simulink model "PID_Gravity"  (R2024a)
settings: Solver=FixedStepAuto  StartTime=0.0  StopTime=10.0  FixedStep=1e-5  RelTol=1e-3
settings Model: Creator=erhan  LastModifiedBy=erhan

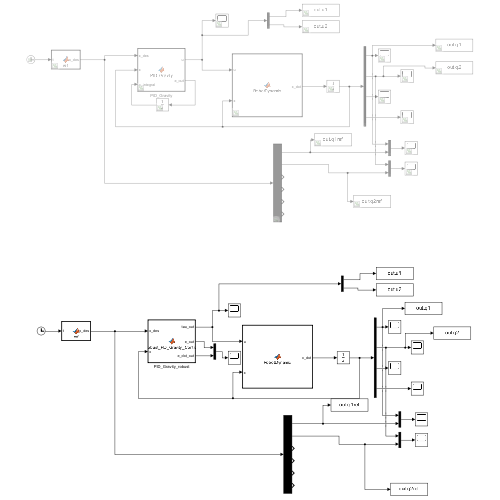
[thumbnail: Simulink's stored preview of the top-level diagram]
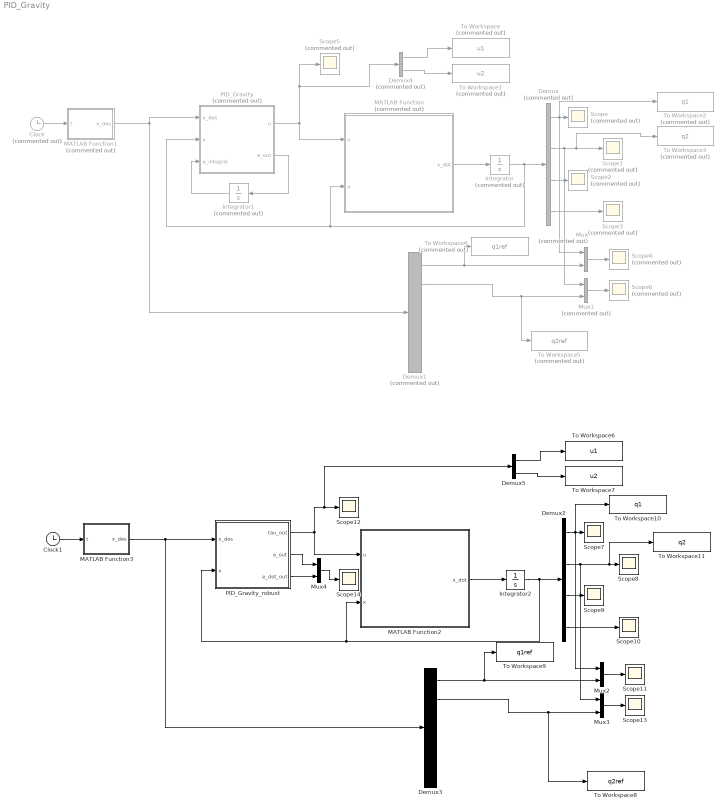
== system PID_Gravity ==
  Clock : Clock  Commented=on
  Clock1 : Clock
  Demux : Demux  Commented=on
  Demux1 : Demux  Commented=on  Outputs=6
  Demux2 : Demux
  Demux3 : Demux  Outputs=6
  Demux4 : Demux  Commented=on  Outputs=2
  Demux5 : Demux  Outputs=2
  Integrator : Integrator  Commented=on  InitialCondition=[0;0;0;0]
  Integrator1 : Integrator  Commented=on  InitialCondition=[0;0]
  Integrator2 : Integrator  InitialCondition=[0;0;0;0]
  MATLAB Function : MATLAB Function  Commented=on  TreatAsAtomicUnit=on
  MATLAB Function1 : MATLAB Function  Commented=on  TreatAsAtomicUnit=on
  MATLAB Function2 : MATLAB Function  TreatAsAtomicUnit=on
  MATLAB Function3 : MATLAB Function  TreatAsAtomicUnit=on
  Mux : Mux  Commented=on  Inputs=2
  Mux1 : Mux  Commented=on  Inputs=2
  Mux2 : Mux  Inputs=2
  Mux3 : Mux  Inputs=2
  Mux4 : Mux  Inputs=2
  PID_Gravity : MATLAB Function  Commented=on  TreatAsAtomicUnit=on
  PID_Gravity_robust : MATLAB Function  TreatAsAtomicUnit=on
  Scope{,1..6} (7 alike) : Scope  Commented=on
  Scope{7..14} (8 alike) : Scope
  To Workspace : ToWorkspace  Commented=on  VariableName=u1  SaveFormat=Timeseries  SampleTime=-1
  To Workspace1 : ToWorkspace  Commented=on  VariableName=u2  SaveFormat=Timeseries  SampleTime=-1
  To Workspace10 : ToWorkspace  VariableName=q1  SaveFormat=Timeseries  SampleTime=-1
  To Workspace11 : ToWorkspace  VariableName=q2  SaveFormat=Timeseries  SampleTime=-1
  To Workspace2 : ToWorkspace  Commented=on  VariableName=q1  SaveFormat=Timeseries  SampleTime=-1
  To Workspace3 : ToWorkspace  Commented=on  VariableName=q2  SaveFormat=Timeseries  SampleTime=-1
  To Workspace4 : ToWorkspace  Commented=on  VariableName=q1ref  SaveFormat=Timeseries  SampleTime=-1
  To Workspace5 : ToWorkspace  Commented=on  VariableName=q2ref  SaveFormat=Timeseries  SampleTime=-1
  To Workspace6 : ToWorkspace  VariableName=u1  SaveFormat=Timeseries  SampleTime=-1
  To Workspace7 : ToWorkspace  VariableName=u2  SaveFormat=Timeseries  SampleTime=-1
  To Workspace8 : ToWorkspace  VariableName=q2ref  SaveFormat=Timeseries  SampleTime=-1
  To Workspace9 : ToWorkspace  VariableName=q1ref  SaveFormat=Timeseries  SampleTime=-1
  wires:
  MATLAB Function/1(x_dot) -> Integrator/1
  Integrator/1 -> Demux/1, PID_Gravity/2(x), MATLAB Function/2(x)
  Demux/1 -> To Workspace2/1, Mux/1, Scope/1
  Demux/2 -> To Workspace3/1, Scope1/1, Mux1/1
  Demux/3 -> Scope2/1
  Demux/4 -> Scope3/1
  PID_Gravity/1(u) -> MATLAB Function/1(u), Demux4/1, Scope5/1
  MATLAB Function1/1(x_des) -> Demux1/1, PID_Gravity/1(x_des)
  Clock/1 -> MATLAB Function1/1(t)
  Mux/1 -> Scope4/1
  Demux1/1 -> To Workspace4/1, Mux/2
  Demux1/2 -> To Workspace5/1, Mux1/2
  Mux1/1 -> Scope6/1
  PID_Gravity/2(e_out) -> Integrator1/1
  Integrator1/1 -> PID_Gravity/3(e_integral)
  Mux3/1 -> Scope13/1
  Demux3/1 -> To Workspace9/1, Mux2/2
  Mux2/1 -> Scope11/1
  Clock1/1 -> MATLAB Function3/1(t)
  MATLAB Function3/1(x_des) -> PID_Gravity_robust/1(x_des), Demux3/1
  PID_Gravity_robust/1(tau_out) -> MATLAB Function2/1(u), Demux5/1, Scope12/1
  Demux2/4 -> Scope10/1
  Demux2/3 -> Scope9/1
  Demux2/2 -> Mux3/1, To Workspace11/1, Scope8/1
  Demux2/1 -> To Workspace10/1, Scope7/1, Mux2/1
  Integrator2/1 -> MATLAB Function2/2(x), PID_Gravity_robust/2(x), Demux2/1
  MATLAB Function2/1(x_dot) -> Integrator2/1
  PID_Gravity_robust/2(e_out) -> Mux4/1
  PID_Gravity_robust/3(e_dot_out) -> Mux4/2
  Mux4/1 -> Scope14/1
  Demux4/1 -> To Workspace/1
  Demux4/2 -> To Workspace1/1
  Demux3/2 -> To Workspace8/1, Mux3/2
  Demux5/2 -> To Workspace7/1
  Demux5/1 -> To Workspace6/1

== matlab function PID_Gravity/PID_Gravity ==
  data: x_des input; u output; x input; e_integral input; e_out output
function [u, e_out] = PID_Gravity(x_des, x, e_integral)
% GİRİŞLER:
% x_des     : [6x1] (qd1, qd2, dqd1, dqd2, ddqd1, ddqd2)
% x         : [4x1] (q1, q2, dq1, dq2)
% e_integral: [2x1] (Hatanın İntegrali - Simulink Integrator bloğundan gelecek)

% ÇIKIŞLAR:
% u     : [2x1] Torklar
% e_out : [2x1] Anlık Hata (Bunu dışarıda Integrate edeceksiniz)

% --- PARAMETRELER ---
m1=1; m2=1;
L1=1; L2=1;
g=9.81;

% Kazançlar
Kp = 100;
Kd = 50;
Ki = 1; % İntegral Kazancı

% --- SİNYALLERİ AYRIŞTIRMA ---
qd   = x_des(1:2);   % Hedef Pozisyon
qdp  = x_des(3:4);   % Hedef Hız


q_act  = x(1:2);     % Gerçek Pozisyon
dq_act = x(3:4);     % Gerçek Hız

% --- HATA HESABI ---
e  = qd - q_act;      % Konum Hatası
ep = qdp - dq_act;    % Hız Hatası

% İntegral için dışarıya hata gönderiyoruz
e_out = e; 

% --- DİNAMİK MATRİSLER (Uniform Rod Model) ---
% M (Atalet) Matrisi


% C (Coriolis/Merkezkaç) Vektörü


% G (Yerçekimi) Vektörü
G1 = (g*(L2*m2*cos(q_act(1) + q_act(2)) + L1*m1*cos(q_act(1)) + 2*L1*m2*cos(q_act(1))))/2;
G2 = (L2*g*m2*cos(q_act(1) + q_act(2)))/2;

% N (Nonlinear Terms)


% --- KONTROL YASASI (PID) ---
% s (Sanal İvme) = ddqd + Kd*de + Kp*e + Ki*integral(e)
s1 = Kd*ep(1) + Kp*e(1) + Ki*e_integral(1);
s2 = Kd*+ep(2) + Kp*e(2) + Ki*e_integral(2);
tau1 = s1+G1;
tau2 = s2+G2;


u = [tau1; tau2];

end

== matlab function PID_Gravity/MATLAB Function ==
  data: u input; x_dot output; x input
function x_dot = RobotDynamic(u,x)
% Parametreler
m1=1;
m2=1;
L1=1;
L2=1;
g=9.81;

% --- M (Atalet) Matrisi ---
M11 = (L1^2*m1)/3 + L1^2*m2 + (L2^2*m2)/3 + L1*L2*m2*cos(x(2));
M12 = (L2*m2*(2*L2 + 3*L1*cos(x(2))))/6;
M21 = M12;
M22 = (L2^2*m2)/3;

% --- C (Coriolis/Merkezkaç) Vektörü ---
C1 = -(L1*L2*x(3)*m2*sin(x(2))*(2*x(3) + x(4)))/2;
C2 = (L1*L2*x(3)^2*m2*sin(x(2)))/2;

% --- G (Yerçekimi) Vektörü ---
G1 = (g*(L2*m2*cos(x(1) + x(2)) + L1*m1*cos(x(1)) + 2*L1*m2*cos(x(1))))/2;
G2 = (L2*g*m2*cos(x(1) + x(2)))/2;


% N (Nonlinear Terms)
N1 = G1 + C1;
N2 = G2 + C2;

% --- MATRİS TERSİ (Inverse Matrix) HESABI ---
% Determinant
det = M11*M22 - M12*M21;

% HATA BURADAYDI (Düzeltildi)
MI11 = M22/det;
MI12 = -M12/det;
MI21 = -M21/det;  % Eksikti, eklendi.
MI22 = M11/det;   % MI11 yerine MI22 yazildi.

% Giriş Torkları
tau1 = u(1);
tau2 = u(2);

% --- İVMELERİN HESAPLANMASI ---
% Denklem: ddq = inv(M) * (tau - N)
% q(3) -> ddq1
% q(4) -> ddq2

q = zeros(4,1);
q(1) = x(3); % dq1
q(2) = x(4); % dq2

% Matris çarpımı (Manuel):
% ddq1 = MI11*(tau1 - N1) + MI12*(tau2 - N2)
q(3) = MI11*(tau1 - N1) + MI12*(tau2 - N2);

% ddq2 = MI21*(tau1 - N1) + MI22*(tau2 - N2)
q(4) = MI21*(tau1 - N1) + MI22*(tau2 - N2);

x_dot = q;
end

== matlab function PID_Gravity/MATLAB Function1 ==
  data: t input; x_des output
function x_des = ref(t)


period = 2;
% amp1 = 0.1;
% amp2 = 0.1;
fact = 2*pi/period;
% sinf = sin(fact*t);
% cosf = cos(fact*t);
qd = [0.1 0.1];
qdp = fact*[0 0];
qdpp = -fact^2*qd;
x_des = [qd qdp qdpp]';

end

== matlab function PID_Gravity/MATLAB Function2 ==
  data: u input; x_dot output; x input
function x_dot = RobotDynamic(u,x)
% Parametreler
m1=0.8; m2=2.3;
L1=1; L2=1;
g=9.81;

% --- M (Atalet) Matrisi ---
M11 = (m2*(2*L1^2 + 2*L2^2 + 4*L1*L2*cos(x(2))))/2 + L1^2*m1;
M12 = L2*m2*(L2 + L1*cos(x(2)));
M21 = M12;
M22 = L2^2*m2;

% --- C (Coriolis/Merkezkaç) Vektörü ---
C1 = -L1*L2*x(4)*m2*sin(x(2))*(2*x(3) + x(4));
C2 = L1*L2*x(3)^2*m2*sin(x(2));

% --- G (Yerçekimi) Vektörü ---
G1 = g*m2*(L2*cos(x(1) + x(2)) + L1*cos(x(1))) + L1*g*m1*cos(x(1));
G2 = L2*g*m2*cos(x(1) + x(2));


% N (Nonlinear Terms)
N1 = G1 + C1;
N2 = G2 + C2;

% --- MATRİS TERSİ (Inverse Matrix) HESABI ---
% Determinant
det = M11*M22 - M12*M21;

% HATA BURADAYDI (Düzeltildi)
MI11 = M22/det;
MI12 = -M12/det;
MI21 = -M21/det;  % Eksikti, eklendi.
MI22 = M11/det;   % MI11 yerine MI22 yazildi.

% Giriş Torkları
tau1 = u(1);
tau2 = u(2);

% --- İVMELERİN HESAPLANMASI ---
% Denklem: ddq = inv(M) * (tau - N)
% q(3) -> ddq1
% q(4) -> ddq2

q = zeros(4,1);
q(1) = x(3); % dq1
q(2) = x(4); % dq2

% Matris çarpımı (Manuel):
% ddq1 = MI11*(tau1 - N1) + MI12*(tau2 - N2)
q(3) = MI11*(tau1 - N1) + MI12*(tau2 - N2);

% ddq2 = MI21*(tau1 - N1) + MI22*(tau2 - N2)
q(4) = MI21*(tau1 - N1) + MI22*(tau2 - N2);

x_dot = q;
end

== matlab function PID_Gravity/MATLAB Function3 ==
  data: t input; x_des output
function x_des = ref(t)


period = 2;
% amp1 = 0.1;
% amp2 = 0.1;
fact = 2*pi/period;
% sinf = sin(fact*t);
% cosf = cos(fact*t);
qd = [0.1 0.1];
qdp = fact*[0 0];
qdpp = -fact^2*qd;
x_des = [qd qdp qdpp]';

end

== matlab function PID_Gravity/PID_Gravity_robust ==
  data: x_des input; tau_out output; x input; e_out output; e_dot_out output
function [tau_out, e_out, e_dot_out] = Robust_PD_Gravity_Control(x_des, x)

% Robust_PD_Gravity_Control: Robot için sağlam PD yerçekimi kontrolcüsü uygular.
% Bu fonksiyon, kontrol teorisindeki tau = Kv*r + G - v yasasını esas alır.
% Girişler:
% x_des     : [6x1] (qd, qd_dot, qd_dot_dot) vektörü
% x         : [4x1] (q, dq) anlık durum vektörü
% Çıkışlar:
% tau_out   : [2x1] Kontrol Torku Vektörü
% e_out     : [2x1] Anlık Pozisyon Hatası (Simulink'te integral için kullanılır)
% e_dot_out : [2x1] Anlık Hız Hatası

%% --- PARAMETRELER VE KAZANÇLAR ---
% Kol Parametreleri (m1, m2, a1, a2)
m1 = 0.8; m2 = 2.3;             %
a1 = 1; a2 = 1; g = 9.8;        %

% Kontrol Kazançları ve Filtreleme
Kv = 50 * eye(2);               % Hız Kazanç Matrisi (Kd = Kv)
lam = 1 * eye(2);               % Filtreleme Matrisi (Lambda)
eps = 0.1;                      % Sınırlayıcı Katman Genişliği (epsilon)

%% --- SİNYALLERİ AYRIŞTIRMA ---
qd   = x_des(1:2, 1);           % İstenen Pozisyon (q_d)
qdp  = x_des(3:4, 1);           % İstenen Hız (dq_d)
qdpp = x_des(5:6, 1);           % İstenen İvme (ddq_d)

q_curr = x(1:2, 1);             % Anlık Pozisyon (q)
dq_curr = x(3:4, 1);            % Anlık Hız (dq)

%% --- HATA HESABI ---
e  = qd - q_curr;               % Pozisyon Hatası
ep = qdp - dq_curr;             % Hız Hatası
r = ep + lam * e;               % Filtrelenmiş Hata Vektörü (r)

% İntegral ve Türev için dışarıya gönderilen hatalar
e_out = e; 
e_dot_out = ep;

%% --- SINIRLAYICI FONKSİYON (F) HESABI ---
% mu2: Atalet üst sınırı (Teorik olarak doğru formül)
mu2 = (m1 + m2) * a1^2 + 2 * m2 * a2^2 + 3 * m2 * a1 * a2; 
% nu_B: Coriolis üst sınırı (nu_B)
vB = m2 * a1 * a2; 

% İstenilen İvme ve Hızlar ile filtrelenmiş hata terimleri
f_sig = qdp + lam * e;
f_sig_p = qdpp + lam * ep; 

% F: Toplam belirsizliği sınırlayan fonksiyon (F(x))
F = mu2 * norm(f_sig_p) + vB * norm(dq_curr) * norm(f_sig); 
% Not: İkinci terimde norm([x(3) x(4)]') = norm(dq_curr) kullanıldı.

%% --- KONTROL TORKU (tau) HESABI ---

% 1. G: Yerçekimi Vektörü (G(q))
% Standart yerçekimi matrisinden alınan doğru formül
G = [((m1 + m2) * g * a1 * cos(q_curr(1)) + m2 * g * a2 * cos(q_curr(1) + q_curr(2))); 
      m2 * g * a2 * cos(q_curr(1) + q_curr(2))]; 


div = max([norm(r); eps]); 
v = -r * F / div; 


tau_out = Kv * r + G - v; 

end
